simulink model "FDM"  (R2020b)
settings: Solver=VariableStepAuto  StartTime=0.0  StopTime=t_final  MaxStep=0.1  RelTol=1e-3
values from neighbouring files (symbols this model uses):
  c =     [FDM_N_3.mat]    (also in FDM_N_50.mat; output_C_10.m = evalin('base','c'); output_C_100.m = evalin('base','c'); output_C_3.m = evalin('base','c'))
  initial_100_n = [0.0124453454776 0.0124453454776 0.0124453454776 0.0124453454776 0.0124453454776 0.0124453454776 0.0124453454776 0.0124453454776 0.0124453454776 0.0124453454776 0.0124453454776 0.0124453454776 ... (99 elements, 1x99)]    [FDM_N_3.mat]    (also in FDM_N_50.mat; RUn_Model_FDM.m = repmat(C_avg_n, 1, 99))
  initial_100_p = [0.00900837 0.00900837 0.00900837 0.00900837 0.00900837 0.00900837 0.00900837 0.00900837 0.00900837 0.00900837 0.00900837 0.00900837 ... (99 elements, 1x99)]    [FDM_N_3.mat]    (also in FDM_N_50.mat; RUn_Model_FDM.m = repmat(C_avg_p, 1, 99))
  initial_10_n = [0.0124453454776 0.0124453454776 0.0124453454776 0.0124453454776 0.0124453454776 0.0124453454776 0.0124453454776 0.0124453454776 0.0124453454776]    [FDM_N_3.mat]    (also in FDM_N_50.mat; RUn_Model_FDM.m = repmat(C_avg_n, 1, 9))
  initial_10_p = [0.00900837 0.00900837 0.00900837 0.00900837 0.00900837 0.00900837 0.00900837 0.00900837 0.00900837]    [FDM_N_3.mat]    (also in FDM_N_50.mat; RUn_Model_FDM.m = repmat(C_avg_p, 1, 9))
  initial_3_n = [0.0124453454776 0.0124453454776]    [FDM_N_3.mat]    (also in FDM_N_50.mat; RUn_Model_FDM.m = repmat(C_avg_n, 1, 2))
  initial_3_p = [0.00900837 0.00900837]    [FDM_N_3.mat]    (also in FDM_N_50.mat; RUn_Model_FDM.m = repmat(C_avg_p, 1, 2))
  initial_50_n = [0.0124453454776 0.0124453454776 0.0124453454776 0.0124453454776 0.0124453454776 0.0124453454776 0.0124453454776 0.0124453454776 0.0124453454776 0.0124453454776 0.0124453454776 0.0124453454776 ... (49 elements, 1x49)]    [FDM_N_3.mat]    (also in FDM_N_50.mat; RUn_Model_FDM.m = repmat(C_avg_n, 1, 49))
  initial_50_p = [0.00900837 0.00900837 0.00900837 0.00900837 0.00900837 0.00900837 0.00900837 0.00900837 0.00900837 0.00900837 0.00900837 0.00900837 ... (49 elements, 1x49)]    [FDM_N_3.mat]    (also in FDM_N_50.mat; RUn_Model_FDM.m = repmat(C_avg_p, 1, 49))
  initial_5_n = [0.0124453454776 0.0124453454776 0.0124453454776 0.0124453454776]    [FDM_N_3.mat]    (also in FDM_N_50.mat; RUn_Model_FDM.m = repmat(C_avg_n, 1, 4))
  initial_5_p = [0.00900837 0.00900837 0.00900837 0.00900837]    [FDM_N_3.mat]    (also in FDM_N_50.mat; RUn_Model_FDM.m = repmat(C_avg_p, 1, 4))
settings Model: Creator=moonjihoon  LastModifiedBy=moonjihoon

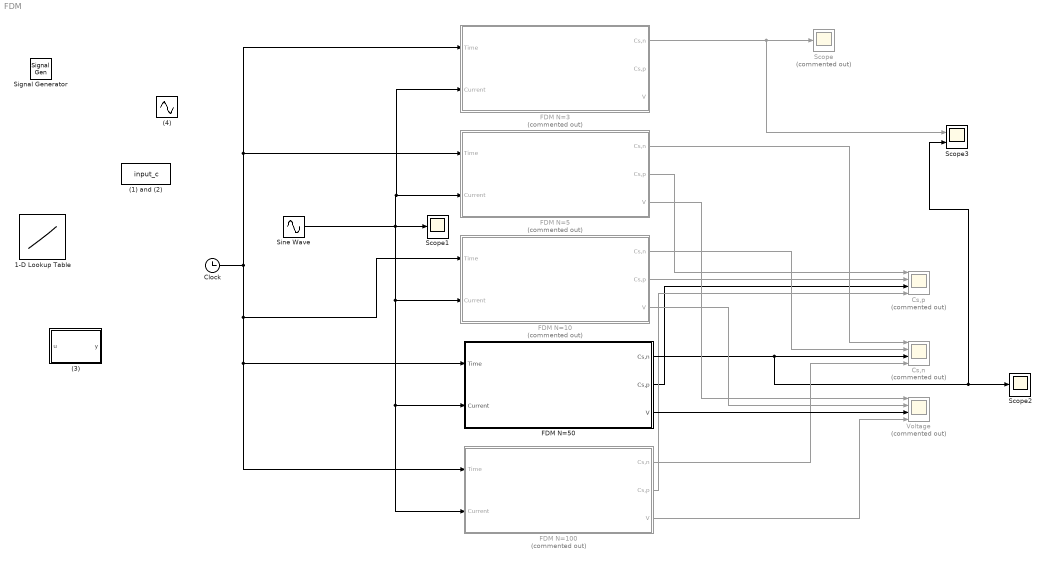
== system FDM ==
  (1) and (2) : MATLABFcn  MATLABFcn=input_c
  (3) : MATLAB Function  TreatAsAtomicUnit=on
  (4) : Sin  Amplitude=10  Frequency=0.005  Phase=3*pi/2  SampleTime=0
  1-D Lookup Table : Lookup_n-D  NumberOfTableDimensions=1  BreakpointsForDimension1=t  Table=u  InternalRulePriority=Speed  RndMeth=Simplest  InputSameDT=on
  Clock : Clock
  Cs,n : Scope  Commented=on  NumInputPorts=4
  Cs,p : Scope  Commented=on  NumInputPorts=4
  "FDM N=10 " : Subsystem  Commented=on
  FDM N=100 : Subsystem  Commented=on
  FDM N=3 : Subsystem  Commented=on
  FDM N=5 : Subsystem  Commented=on
  "FDM N=50 " : Subsystem
  Scope : Scope  Commented=on
  Scope1 : Scope
  Scope2 : Scope
  Scope3 : Scope  NumInputPorts=2
  Signal Generator : SignalGenerator  WaveForm=square  Amplitude=-4  Frequency=0.006  Units=rad/sec
  Sine Wave : Sin  Amplitude=10  Frequency=0.005  SampleTime=0
  Voltage : Scope  Commented=on  NumInputPorts=4
  wires:
  Sine Wave/1 -> FDM N=3/2(Current), FDM N=5/2(Current), FDM N=100/2(Current), "FDM N=50 "/2(Current), "FDM N=10 "/2(Current), Scope1/1
  FDM N=5/2(Cs,p) -> Cs,p/1
  "FDM N=10 "/2(Cs,p) -> Cs,p/2
  "FDM N=50 "/2(Cs,p) -> Cs,p/3
  FDM N=100/2(Cs,p) -> Cs,p/4
  FDM N=5/1(Cs,n) -> Cs,n/1
  "FDM N=10 "/1(Cs,n) -> Cs,n/2
  "FDM N=50 "/1(Cs,n) -> Scope3/2, Scope2/1, Cs,n/3
  FDM N=100/1(Cs,n) -> Cs,n/4
  FDM N=5/3(V) -> Voltage/1
  "FDM N=10 "/3(V) -> Voltage/2
  "FDM N=50 "/3(V) -> Voltage/3
  FDM N=100/3(V) -> Voltage/4
  FDM N=3/1(Cs,n) -> Scope3/1, Scope/1
  Clock/1 -> "FDM N=10 "/1(Time), "FDM N=50 "/1(Time), FDM N=100/1(Time), FDM N=5/1(Time), FDM N=3/1(Time)

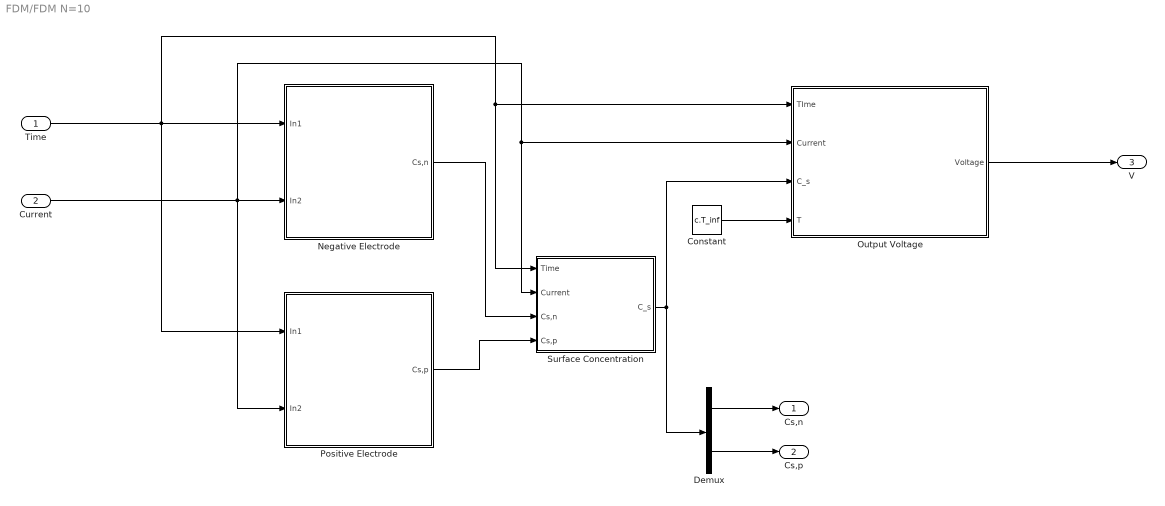
== system FDM/FDM N=10  ==
  Time : Inport
  Current : Inport  Port=2
  Constant : Constant  Value=c.T_inf
  Demux : Demux  Outputs=2
  Negative Electrode : Subsystem
  Output Voltage : Subsystem
  Positive Electrode : Subsystem
  Surface Concentration : Subsystem
  Cs,n : Outport
  Cs,p : Outport  Port=2
  V : Outport  Port=3
  wires:
  Time/1 -> Surface Concentration/1(Time), Output Voltage/1(TIme), Positive Electrode/1(In1), Negative Electrode/1(In1)
  Current/1 -> Surface Concentration/2(Current), Output Voltage/2(Current), Positive Electrode/2(In2), Negative Electrode/2(In2)
  Constant/1 -> Output Voltage/4(T)
  Output Voltage/1(Voltage) -> V/1
  Surface Concentration/1(C_s) -> Output Voltage/3(C_s), Demux/1
  Negative Electrode/1(Cs,n) -> Surface Concentration/3(Cs,n)
  Positive Electrode/1(Cs,p) -> Surface Concentration/4(Cs,p)
  Demux/2 -> Cs,p/1
  Demux/1 -> Cs,n/1

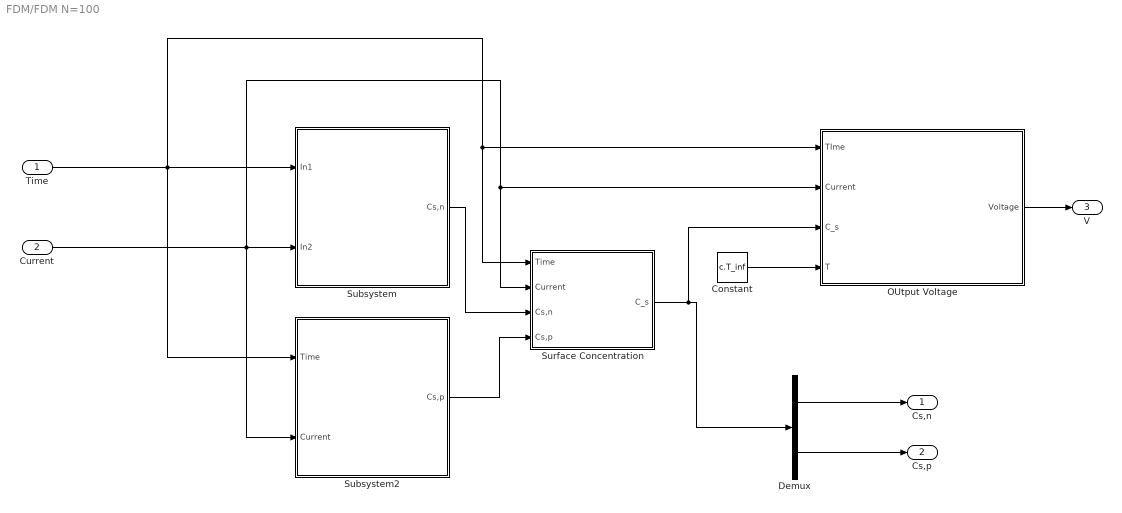
== system FDM/FDM N=100 ==
  Time : Inport
  Current : Inport  Port=2
  Constant : Constant  Value=c.T_inf
  Demux : Demux  Outputs=2
  OUtput Voltage : Subsystem
  Subsystem : Subsystem
  Subsystem2 : Subsystem
  Surface Concentration : Subsystem
  Cs,n : Outport
  Cs,p : Outport  Port=2
  V : Outport  Port=3
  wires:
  Time/1 -> Surface Concentration/1(Time), OUtput Voltage/1(TIme), Subsystem2/1(Time), Subsystem/1(In1)
  Current/1 -> Subsystem2/2(Current), Surface Concentration/2(Current), OUtput Voltage/2(Current), Subsystem/2(In2)
  Constant/1 -> OUtput Voltage/4(T)
  OUtput Voltage/1(Voltage) -> V/1
  Subsystem/1(Cs,n) -> Surface Concentration/3(Cs,n)
  Subsystem2/1(Cs,p) -> Surface Concentration/4(Cs,p)
  Demux/2 -> Cs,p/1
  Demux/1 -> Cs,n/1
  Surface Concentration/1(C_s) -> OUtput Voltage/3(C_s), Demux/1

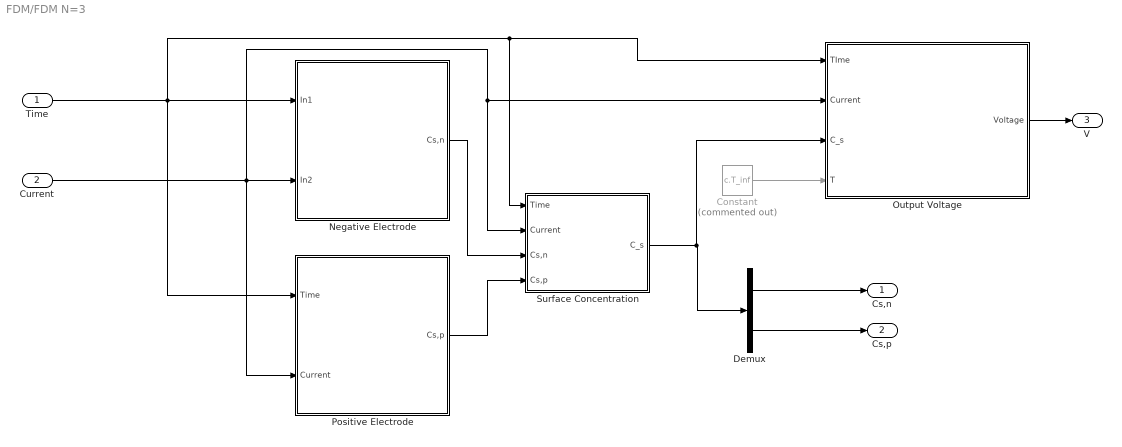
== system FDM/FDM N=3 ==
  Time : Inport
  Current : Inport  Port=2
  Constant : Constant  Commented=on  Value=c.T_inf
  Demux : Demux  Outputs=2
  Negative Electrode : Subsystem
  Output Voltage : Subsystem
  Positive Electrode : Subsystem
  Surface Concentration : Subsystem
  Cs,n : Outport
  Cs,p : Outport  Port=2
  V : Outport  Port=3
  wires:
  Current/1 -> Positive Electrode/2(Current), Surface Concentration/2(Current), Output Voltage/2(Current), Negative Electrode/2(In2)
  Time/1 -> Surface Concentration/1(Time), Output Voltage/1(TIme), Positive Electrode/1(Time), Negative Electrode/1(In1)
  Constant/1 -> Output Voltage/4(T)
  Output Voltage/1(Voltage) -> V/1
  Demux/2 -> Cs,p/1
  Surface Concentration/1(C_s) -> Output Voltage/3(C_s), Demux/1
  Negative Electrode/1(Cs,n) -> Surface Concentration/3(Cs,n)
  Positive Electrode/1(Cs,p) -> Surface Concentration/4(Cs,p)
  Demux/1 -> Cs,n/1

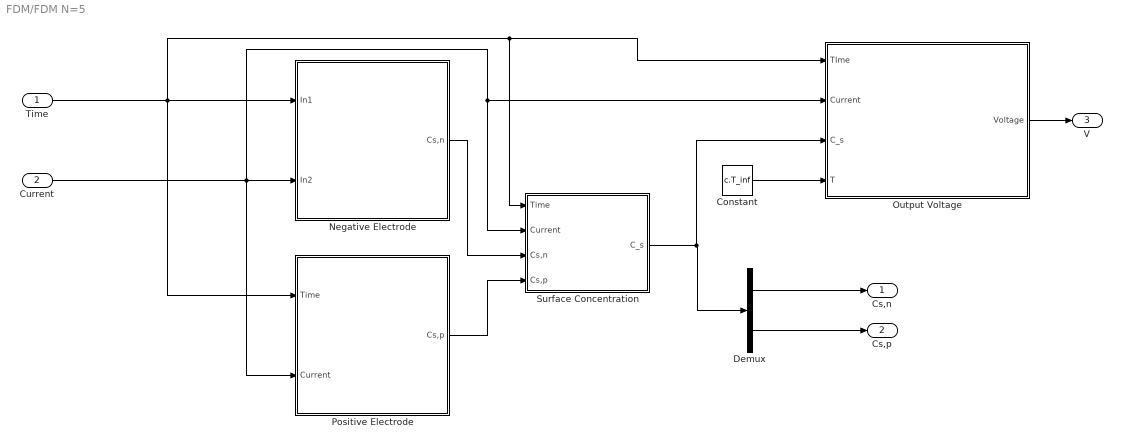
== system FDM/FDM N=5 ==
  Time : Inport
  Current : Inport  Port=2
  Constant : Constant  Value=c.T_inf
  Demux : Demux  Outputs=2
  Negative Electrode : Subsystem
  Output Voltage : Subsystem
  Positive Electrode : Subsystem
  Surface Concentration : Subsystem
  Cs,n : Outport
  Cs,p : Outport  Port=2
  V : Outport  Port=3
  wires:
  Current/1 -> Positive Electrode/2(Current), Surface Concentration/2(Current), Output Voltage/2(Current), Negative Electrode/2(In2)
  Time/1 -> Surface Concentration/1(Time), Output Voltage/1(TIme), Positive Electrode/1(Time), Negative Electrode/1(In1)
  Constant/1 -> Output Voltage/4(T)
  Output Voltage/1(Voltage) -> V/1
  Demux/1 -> Cs,n/1
  Demux/2 -> Cs,p/1
  Surface Concentration/1(C_s) -> Output Voltage/3(C_s), Demux/1
  Negative Electrode/1(Cs,n) -> Surface Concentration/3(Cs,n)
  Positive Electrode/1(Cs,p) -> Surface Concentration/4(Cs,p)

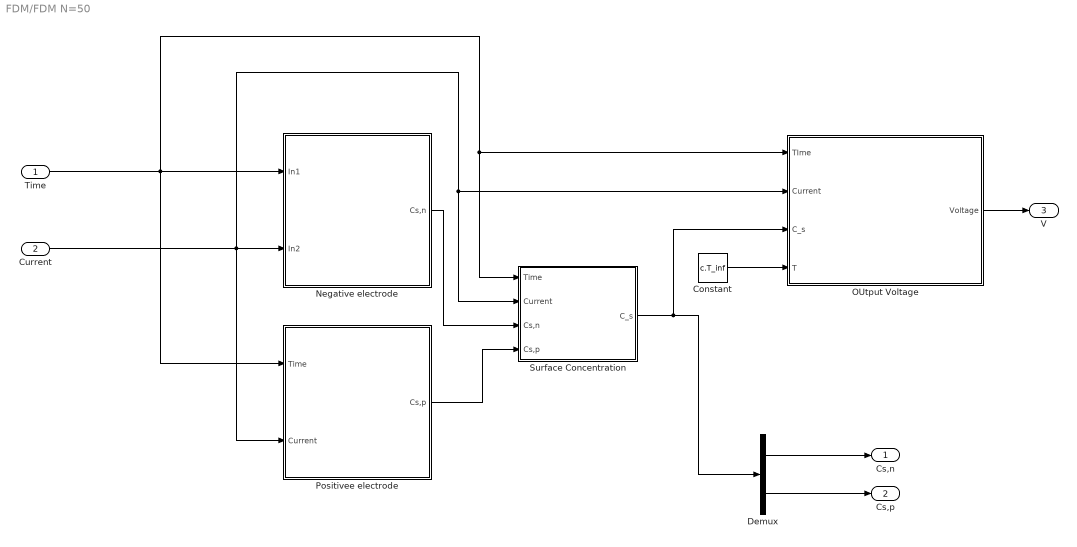
== system FDM/FDM N=50  ==
  Time : Inport
  Current : Inport  Port=2
  Constant : Constant  Value=c.T_inf
  Demux : Demux  Outputs=2
  Negative electrode : Subsystem
  OUtput Voltage : Subsystem
  Positivee electrode : Subsystem
  Surface Concentration : Subsystem
  Cs,n : Outport
  Cs,p : Outport  Port=2
  V : Outport  Port=3
  wires:
  Time/1 -> Surface Concentration/1(Time), OUtput Voltage/1(TIme), Positivee electrode/1(Time), Negative electrode/1(In1)
  Current/1 -> Positivee electrode/2(Current), Surface Concentration/2(Current), OUtput Voltage/2(Current), Negative electrode/2(In2)
  Constant/1 -> OUtput Voltage/4(T)
  OUtput Voltage/1(Voltage) -> V/1
  Negative electrode/1(Cs,n) -> Surface Concentration/3(Cs,n)
  Positivee electrode/1(Cs,p) -> Surface Concentration/4(Cs,p)
  Demux/1 -> Cs,n/1
  Demux/2 -> Cs,p/1
  Surface Concentration/1(C_s) -> OUtput Voltage/3(C_s), Demux/1

== system FDM/FDM N=10 /Negative Electrode ==
  In1 : Inport
  In2 : Inport  Port=2
  Integrator : Integrator  InitialCondition=initial_10_n
  Interpreted MATLAB Function : MATLABFcn  MATLABFcn=state_eqns_fdm_10
  Mux : Mux  Inputs=3
  Cs,n : Outport
  wires:
  Interpreted MATLAB Function/1 -> Integrator/1
  In1/1 -> Mux/1
  In2/1 -> Mux/2
  Mux/1 -> Interpreted MATLAB Function/1
  Integrator/1 -> Cs,n/1, Mux/3

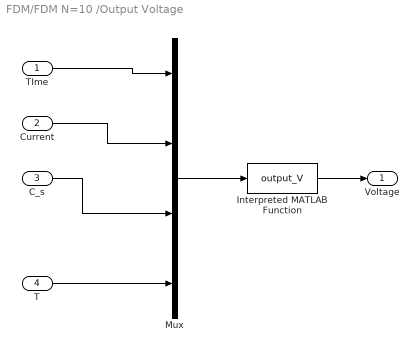
== system FDM/FDM N=10 /Output Voltage ==
  TIme : Inport
  Current : Inport  Port=2
  C_s : Inport  Port=3
  T : Inport  Port=4
  Interpreted MATLAB Function : MATLABFcn  MATLABFcn=output_V
  Mux : Mux
  Voltage : Outport
  wires:
  TIme/1 -> Mux/1
  Interpreted MATLAB Function/1 -> Voltage/1
  Mux/1 -> Interpreted MATLAB Function/1
  Current/1 -> Mux/2
  C_s/1 -> Mux/3
  T/1 -> Mux/4

== system FDM/FDM N=10 /Positive Electrode ==
  In1 : Inport
  In2 : Inport  Port=2
  Integrator : Integrator  InitialCondition=initial_10_p
  Interpreted MATLAB Function : MATLABFcn  MATLABFcn=state_eqns_fdm_10p
  Mux : Mux  Inputs=3
  Cs,p : Outport
  wires:
  Interpreted MATLAB Function/1 -> Integrator/1
  In1/1 -> Mux/1
  In2/1 -> Mux/2
  Mux/1 -> Interpreted MATLAB Function/1
  Integrator/1 -> Cs,p/1, Mux/3

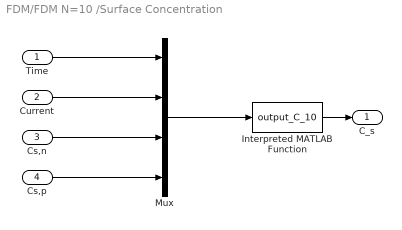
== system FDM/FDM N=10 /Surface Concentration ==
  Time : Inport
  Current : Inport  Port=2
  Cs,n : Inport  Port=3
  Cs,p : Inport  Port=4
  Interpreted MATLAB Function : MATLABFcn  MATLABFcn=output_C_10
  Mux : Mux
  C_s : Outport
  wires:
  Interpreted MATLAB Function/1 -> C_s/1
  Time/1 -> Mux/1
  Current/1 -> Mux/2
  Cs,n/1 -> Mux/3
  Mux/1 -> Interpreted MATLAB Function/1
  Cs,p/1 -> Mux/4

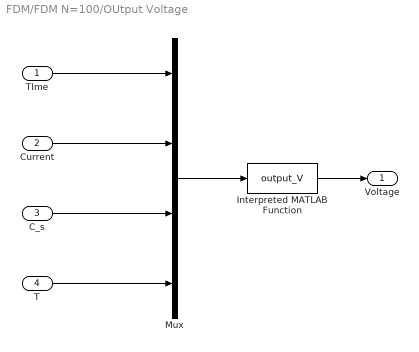
== system FDM/FDM N=100/OUtput Voltage ==
  TIme : Inport
  Current : Inport  Port=2
  C_s : Inport  Port=3
  T : Inport  Port=4
  Interpreted MATLAB Function : MATLABFcn  MATLABFcn=output_V
  Mux : Mux
  Voltage : Outport
  wires:
  TIme/1 -> Mux/1
  Interpreted MATLAB Function/1 -> Voltage/1
  Mux/1 -> Interpreted MATLAB Function/1
  Current/1 -> Mux/2
  C_s/1 -> Mux/3
  T/1 -> Mux/4

== system FDM/FDM N=100/Subsystem ==
  In1 : Inport
  In2 : Inport  Port=2
  Integrator : Integrator  InitialCondition=initial_100_n
  Interpreted MATLAB Function : MATLABFcn  MATLABFcn=state_eqns_fdm_100
  Mux : Mux  Inputs=3
  Cs,n : Outport
  wires:
  Interpreted MATLAB Function/1 -> Integrator/1
  In1/1 -> Mux/1
  In2/1 -> Mux/2
  Mux/1 -> Interpreted MATLAB Function/1
  Integrator/1 -> Cs,n/1, Mux/3

== system FDM/FDM N=100/Subsystem2 ==
  Time : Inport
  Current : Inport  Port=2
  Integrator : Integrator  InitialCondition=initial_100_p
  Interpreted MATLAB Function : MATLABFcn  MATLABFcn=state_eqns_fdm_100p
  Mux : Mux  Inputs=3
  Cs,p : Outport
  wires:
  Interpreted MATLAB Function/1 -> Integrator/1
  Time/1 -> Mux/1
  Current/1 -> Mux/2
  Mux/1 -> Interpreted MATLAB Function/1
  Integrator/1 -> Cs,p/1, Mux/3

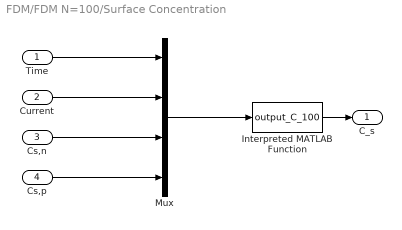
== system FDM/FDM N=100/Surface Concentration ==
  Time : Inport
  Current : Inport  Port=2
  Cs,n : Inport  Port=3
  Cs,p : Inport  Port=4
  Interpreted MATLAB Function : MATLABFcn  MATLABFcn=output_C_100
  Mux : Mux
  C_s : Outport
  wires:
  Interpreted MATLAB Function/1 -> C_s/1
  Time/1 -> Mux/1
  Current/1 -> Mux/2
  Cs,n/1 -> Mux/3
  Mux/1 -> Interpreted MATLAB Function/1
  Cs,p/1 -> Mux/4

== system FDM/FDM N=3/Negative Electrode ==
  In1 : Inport
  In2 : Inport  Port=2
  Integrator : Integrator  InitialCondition=initial_3_n
  Interpreted MATLAB Function : MATLABFcn  MATLABFcn=state_eqns_fdm_3
  Mux : Mux  Inputs=3
  Cs,n : Outport
  wires:
  Interpreted MATLAB Function/1 -> Integrator/1
  In1/1 -> Mux/1
  In2/1 -> Mux/2
  Mux/1 -> Interpreted MATLAB Function/1
  Integrator/1 -> Cs,n/1, Mux/3

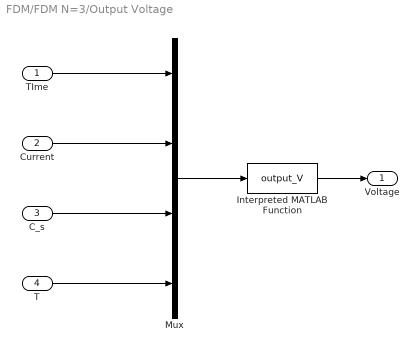
== system FDM/FDM N=3/Output Voltage ==
  TIme : Inport
  Current : Inport  Port=2
  C_s : Inport  Port=3
  T : Inport  Port=4
  Interpreted MATLAB Function : MATLABFcn  MATLABFcn=output_V
  Mux : Mux
  Voltage : Outport
  wires:
  TIme/1 -> Mux/1
  Interpreted MATLAB Function/1 -> Voltage/1
  Mux/1 -> Interpreted MATLAB Function/1
  Current/1 -> Mux/2
  C_s/1 -> Mux/3
  T/1 -> Mux/4

== system FDM/FDM N=3/Positive Electrode ==
  Time : Inport
  Current : Inport  Port=2
  Integrator : Integrator  InitialCondition=initial_3_p
  Interpreted MATLAB Function : MATLABFcn  MATLABFcn=state_eqns_fdm_3p
  Mux : Mux  Inputs=3
  Cs,p : Outport
  wires:
  Interpreted MATLAB Function/1 -> Integrator/1
  Time/1 -> Mux/1
  Current/1 -> Mux/2
  Mux/1 -> Interpreted MATLAB Function/1
  Integrator/1 -> Cs,p/1, Mux/3

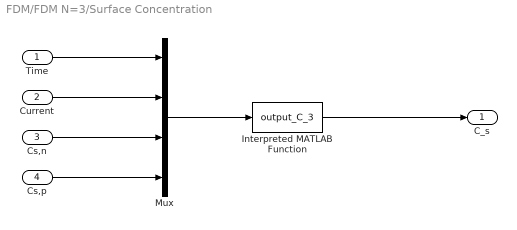
== system FDM/FDM N=3/Surface Concentration ==
  Time : Inport
  Current : Inport  Port=2
  Cs,n : Inport  Port=3
  Cs,p : Inport  Port=4
  Interpreted MATLAB Function : MATLABFcn  MATLABFcn=output_C_3
  Mux : Mux
  C_s : Outport
  wires:
  Time/1 -> Mux/1
  Current/1 -> Mux/2
  Cs,n/1 -> Mux/3
  Mux/1 -> Interpreted MATLAB Function/1
  Cs,p/1 -> Mux/4
  Interpreted MATLAB Function/1 -> C_s/1

== system FDM/FDM N=5/Negative Electrode ==
  In1 : Inport
  In2 : Inport  Port=2
  Integrator : Integrator  InitialCondition=initial_5_n
  Interpreted MATLAB Function : MATLABFcn  MATLABFcn=state_eqns_fdm_5
  Mux : Mux  Inputs=3
  Cs,n : Outport
  wires:
  Interpreted MATLAB Function/1 -> Integrator/1
  In1/1 -> Mux/1
  In2/1 -> Mux/2
  Mux/1 -> Interpreted MATLAB Function/1
  Integrator/1 -> Cs,n/1, Mux/3

== system FDM/FDM N=5/Output Voltage ==
  TIme : Inport
  Current : Inport  Port=2
  C_s : Inport  Port=3
  T : Inport  Port=4
  Interpreted MATLAB Function : MATLABFcn  MATLABFcn=output_V
  Mux : Mux
  Voltage : Outport
  wires:
  TIme/1 -> Mux/1
  Interpreted MATLAB Function/1 -> Voltage/1
  Mux/1 -> Interpreted MATLAB Function/1
  Current/1 -> Mux/2
  C_s/1 -> Mux/3
  T/1 -> Mux/4

== system FDM/FDM N=5/Positive Electrode ==
  Time : Inport
  Current : Inport  Port=2
  Integrator : Integrator  InitialCondition=initial_5_p
  Interpreted MATLAB Function : MATLABFcn  MATLABFcn=state_eqns_fdm_5p
  Mux : Mux  Inputs=3
  Cs,p : Outport
  wires:
  Interpreted MATLAB Function/1 -> Integrator/1
  Time/1 -> Mux/1
  Current/1 -> Mux/2
  Mux/1 -> Interpreted MATLAB Function/1
  Integrator/1 -> Cs,p/1, Mux/3

== system FDM/FDM N=5/Surface Concentration ==
  Time : Inport
  Current : Inport  Port=2
  Cs,n : Inport  Port=3
  Cs,p : Inport  Port=4
  Interpreted MATLAB Function : MATLABFcn  MATLABFcn=output_C_5
  Mux : Mux
  C_s : Outport
  wires:
  Interpreted MATLAB Function/1 -> C_s/1
  Time/1 -> Mux/1
  Current/1 -> Mux/2
  Cs,n/1 -> Mux/3
  Mux/1 -> Interpreted MATLAB Function/1
  Cs,p/1 -> Mux/4

== system FDM/FDM N=50 /Negative electrode ==
  In1 : Inport
  In2 : Inport  Port=2
  Integrator : Integrator  InitialCondition=initial_50_n
  Interpreted MATLAB Function : MATLABFcn  MATLABFcn=state_eqns_fdm_50
  Mux : Mux  Inputs=3
  Cs,n : Outport
  wires:
  Interpreted MATLAB Function/1 -> Integrator/1
  In1/1 -> Mux/1
  In2/1 -> Mux/2
  Mux/1 -> Interpreted MATLAB Function/1
  Integrator/1 -> Cs,n/1, Mux/3

== system FDM/FDM N=50 /OUtput Voltage ==
  TIme : Inport
  Current : Inport  Port=2
  C_s : Inport  Port=3
  T : Inport  Port=4
  Interpreted MATLAB Function : MATLABFcn  MATLABFcn=output_V
  Mux : Mux
  Voltage : Outport
  wires:
  TIme/1 -> Mux/1
  Interpreted MATLAB Function/1 -> Voltage/1
  Mux/1 -> Interpreted MATLAB Function/1
  Current/1 -> Mux/2
  C_s/1 -> Mux/3
  T/1 -> Mux/4

== system FDM/FDM N=50 /Positivee electrode ==
  Time : Inport
  Current : Inport  Port=2
  Integrator : Integrator  InitialCondition=initial_50_p
  Interpreted MATLAB Function : MATLABFcn  MATLABFcn=state_eqns_fdm_50p
  Mux : Mux  Inputs=3
  Cs,p : Outport
  wires:
  Interpreted MATLAB Function/1 -> Integrator/1
  Time/1 -> Mux/1
  Current/1 -> Mux/2
  Mux/1 -> Interpreted MATLAB Function/1
  Integrator/1 -> Cs,p/1, Mux/3

== system FDM/FDM N=50 /Surface Concentration ==
  Time : Inport
  Current : Inport  Port=2
  Cs,n : Inport  Port=3
  Cs,p : Inport  Port=4
  Interpreted MATLAB Function : MATLABFcn  MATLABFcn=output_C_50
  Mux : Mux
  C_s : Outport
  wires:
  Interpreted MATLAB Function/1 -> C_s/1
  Time/1 -> Mux/1
  Current/1 -> Mux/2
  Cs,n/1 -> Mux/3
  Mux/1 -> Interpreted MATLAB Function/1
  Cs,p/1 -> Mux/4

== matlab function FDM/(3) ==
  data: u input; y output
function y = fcn(u)

y = exp(-0.0055*u).*10.*sin(0.02*pi*u);
